simulink library "TurnRight"  (R2018b)
settings: Solver=VariableStepAuto  StartTime=0.0  StopTime=10.0  RelTol=1e-3
settings Model: Creator=billg  LastModifiedBy=Sjoerd

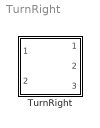
== system TurnRight ==
  TurnRight : Stateflow chart  TreatAsAtomicUnit=on

== stateflow chart TurnRight/TurnRight ==
  state wheels
    state left [parallel]
      settings: executionOrder=1
      state turn90r_lwheel
        entry:
        leftMotor = 20;
        leftOffset = leftEncoder;
      state stop_left
        entry:
        leftMotor = 0;
      (default) -> turn90r_lwheel
      turn90r_lwheel -> stop_left : [(leftEncoder - leftOffset) >= 160]
    state right [parallel]
      settings: executionOrder=2
      state turn90r_rwheel
        entry:
        rightMotor = -20;
        rightOffset = rightEncoder;
      state stop_right
        entry:
        rightMotor = 0;
      (default) -> turn90r_rwheel
      turn90r_rwheel -> stop_right : [(rightOffset - rightEncoder) >= 160]
  state Done
    entry:
    TURN = false;
  (default) -> wheels
  wheels -> Done : [rightMotor ==0 && leftMotor == 0]
  data: leftEncoder input; rightEncoder input; leftMotor output int32 size=1; rightMotor output int32 size=1; leftOffset local; rightOffset local; TURN output boolean size=1
